simulink library "icc_lib_avg_path1_n1"  (R2018b)
settings: Solver=VariableStepAuto  StartTime=0.0  StopTime=10.0  RelTol=1e-3
undefined symbols (not defined in the file or in its folder): icc_lib_avg_path, path1
libraries: simulink x34, simulink_extras x8, $bdroot x2
(part 2 of 4)

== system icc_lib_avg_path1_n1/path_EGM1 ==
  mode1 : Inport
  mode2 : Inport  Port=2
  v1 : Inport  Port=3
  v2 : Inport  Port=4
  "xy1 " : Inport  Port=5
  xy2 : Inport  Port=6
  AND : Logic  IconShape=distinctive  AllPortsSameDT=off  OutDataTypeStr=boolean
  Data Type Conversion : DataTypeConversion  OutDataTypeStr=boolean
  Data Type Conversion1 : DataTypeConversion  OutDataTypeStr=boolean
  Delayed v1 : TransportDelay  DelayTime=0  BufferSize=200704
  Delayed v2 : TransportDelay  DelayTime=0  BufferSize=200704
  Demux : Demux  Outputs=2
  Demux1 : Demux  Outputs=2
  Logical Operator1 : Logic  Operator=OR  AllPortsSameDT=off  OutDataTypeStr=boolean
  Logical Operator2 : Logic  Operator=OR  AllPortsSameDT=off  OutDataTypeStr=boolean
  Mux : Mux  Inputs=6
  Path : Stateflow chart  TreatAsAtomicUnit=on
  Relay switch1 : MultiPortSwitch  DataPortOrder=Zero-based contiguous  Inputs=2  zeroidx=on
  Relay switch2 : MultiPortSwitch  DataPortOrder=Zero-based contiguous  Inputs=2  zeroidx=on
  S-R Flip-Flop : simulink_extras/Flip Flops/S-R Flip-Flop  initial_condition=0
  S-R Flip-Flop1 : simulink_extras/Flip Flops/S-R Flip-Flop  initial_condition=0
  Terminator : Terminator
  Terminator1 : Terminator
  Transport Delay1 : TransportDelay  DelayTime=0.1
  Transport Delay2 : TransportDelay  DelayTime=0.1
  cell1 resting : simulink/Logic and Bit Operations/Compare To Constant  relop===  const=0  OutDataTypeStr=boolean
  cell1FinishR : simulink/Logic and Bit Operations/Compare To Constant  relop=>=  const=1  OutDataTypeStr=boolean
  cell2 resting : simulink/Logic and Bit Operations/Compare To Constant  relop===  const=0  OutDataTypeStr=boolean
  cell2FinishR : simulink/Logic and Bit Operations/Compare To Constant  relop=>=  const=1  OutDataTypeStr=boolean
  cell2FinishR1 : simulink/Logic and Bit Operations/Compare To Constant  relop=~=  const=0  OutDataTypeStr=boolean
  cell2FinishR2 : simulink/Logic and Bit Operations/Compare To Constant  relop=~=  const=4  OutDataTypeStr=boolean
  zero : Constant  Value=-67.6
  zero1 : Constant  Value=-67.6
  relay_1 : Outport
  relay_2 : Outport  Port=2
  egm : Outport  Port=3
  wires:
  Data Type Conversion1/1 -> S-R Flip-Flop1/1
  Data Type Conversion/1 -> S-R Flip-Flop/1
  mode1/1 -> cell1FinishR/1, Transport Delay1/1, Path/1(mode1)
  Transport Delay2/1 -> Path/4(mdelay2), cell2 resting/1
  cell1FinishR/1 -> Logical Operator2/1
  Logical Operator2/1 -> S-R Flip-Flop1/2
  cell2 resting/1 -> Logical Operator2/2
  cell1 resting/1 -> Logical Operator1/2
  AND/1 -> Logical Operator1/1
  Logical Operator1/1 -> S-R Flip-Flop/2
  Relay switch2/1 -> relay_2/1
  S-R Flip-Flop1/2 -> Terminator1/1
  v1/1 -> Delayed v1/1
  Path/1(relay1) -> Data Type Conversion/1
  Delayed v1/1 -> Relay switch1/3
  S-R Flip-Flop1/1 -> Relay switch2/1
  Path/2(relay2) -> Data Type Conversion1/1
  v2/1 -> Delayed v2/1
  zero1/1 -> Relay switch2/2
  zero/1 -> Relay switch1/2
  S-R Flip-Flop/2 -> Terminator/1
  S-R Flip-Flop/1 -> Relay switch1/1
  Relay switch1/1 -> relay_1/1
  Delayed v2/1 -> Relay switch2/3
  mode2/1 -> cell2FinishR2/1, cell2FinishR1/1, Path/3(mode2), Transport Delay2/1
  Transport Delay1/1 -> Path/2(mdelay1), cell1 resting/1
  cell2FinishR1/1 -> AND/2
  cell2FinishR2/1 -> AND/1
  "xy1 "/1 -> Demux/1
  Demux/1 -> [x1]
  Demux/2 -> [y1]
  Mux/1 -> egm/1
  Path/3(t1) -> [t1]
  Path/4(t2) -> [t2]
  [t1] -> Mux/1
  [t2] -> Mux/2
  [x1] -> Mux/3
  [y1] -> Mux/4
  xy2/1 -> Demux1/1
  Demux1/1 -> [x2]
  Demux1/2 -> [y2]
  [y2] -> Mux/6
  [x2] -> Mux/5

== system icc_lib_avg_path1_n1/ICC /ODE ==
  q : Inport
  vreset : Inport  Port=2
  d0 : Inport  Port=3
  d1 : Inport  Port=4
  d2 : Inport  Port=5
  d3 : Inport  Port=6
  reset : Inport  Port=7
  IC : InitialCondition  Value=0
  Memory1 : Memory
  Multiport Switch1 : MultiPortSwitch  DataPortOrder=Zero-based contiguous  Inputs=6  zeroidx=on
  Switch Case : SwitchCase  CaseConditions={0,1,2,3,4,5}  ShowDefaultCase=off
  q0 : Subsystem  TreatAsAtomicUnit=on
  q1 : Subsystem  TreatAsAtomicUnit=on
  q2 : Subsystem  TreatAsAtomicUnit=on
  q3 : Subsystem  TreatAsAtomicUnit=on
  vt_0 : Outport
  wires:
  Multiport Switch1/1 -> Memory1/1
  IC/1 -> [vreset]
  vreset/1 -> IC/1
  reset/1 -> [reset]
  q/1 -> [q]
  q1/1(v) -> [pulse1]
  [q] -> Multiport Switch1/1
  [q] -> Switch Case/1
  [q1] -> q1/Action
  [reset] -> q1/1(reset)
  q2/1(v) -> [v2]
  d2/1 -> q2/3(d)
  [q2] -> q2/Action
  [vreset] -> q2/2(vreset)
  q3/1(v) -> [v3]
  d3/1 -> q3/3(d)
  [reset] -> q3/1(reset)
  [vreset] -> q3/2(vreset)
  q0/1(pulse) -> [v0]
  d0/1 -> q0/3(d)
  [reset] -> q0/1(reset)
  [vreset] -> q0/2(vreset)
  [q3] -> q3/Action
  [q0] -> q0/Action
  Memory1/1 -> vt_0/1
  [v0] -> Multiport Switch1/2
  [pulse1] -> Multiport Switch1/3
  [v2] -> Multiport Switch1/4
  [v3] -> Multiport Switch1/5
  [reset] -> q2/1(reset)
  [vreset] -> q1/2(vreset)
  d1/1 -> q1/3(d)
  Switch Case/1 -> [q0]
  Switch Case/2 -> [q1]
  Switch Case/3 -> [q2]
  Switch Case/4 -> [q3]

== system icc_lib_avg_path1_n1/ICC-multi/ODE ==
  q : Inport
  vreset : Inport  Port=2
  d0 : Inport  Port=3
  d1 : Inport  Port=4
  d2 : Inport  Port=5
  d3 : Inport  Port=6
  reset : Inport  Port=7
  IC : InitialCondition  Value=0
  Memory1 : Memory
  Multiport Switch1 : MultiPortSwitch  DataPortOrder=Zero-based contiguous  Inputs=6  zeroidx=on
  Switch Case : SwitchCase  CaseConditions={0,1,2,3,4,5}  ShowDefaultCase=off
  q0 : Subsystem  TreatAsAtomicUnit=on
  q1 : Subsystem  TreatAsAtomicUnit=on
  q2 : Subsystem  TreatAsAtomicUnit=on
  q3 : Subsystem  TreatAsAtomicUnit=on
  vt_0 : Outport
  wires:
  Switch Case/4 -> [q3]
  Switch Case/3 -> [q2]
  Switch Case/2 -> [q1]
  Switch Case/1 -> [q0]
  d1/1 -> q1/3(d)
  [vreset] -> q1/2(vreset)
  [reset] -> q2/1(reset)
  [v3] -> Multiport Switch1/5
  [v2] -> Multiport Switch1/4
  [pulse1] -> Multiport Switch1/3
  [v0] -> Multiport Switch1/2
  Memory1/1 -> vt_0/1
  [q0] -> q0/Action
  [q3] -> q3/Action
  [vreset] -> q0/2(vreset)
  [reset] -> q0/1(reset)
  d0/1 -> q0/3(d)
  q0/1(pulse) -> [v0]
  [vreset] -> q3/2(vreset)
  [reset] -> q3/1(reset)
  d3/1 -> q3/3(d)
  q3/1(v) -> [v3]
  [vreset] -> q2/2(vreset)
  [q2] -> q2/Action
  d2/1 -> q2/3(d)
  q2/1(v) -> [v2]
  [reset] -> q1/1(reset)
  [q1] -> q1/Action
  [q] -> Switch Case/1
  [q] -> Multiport Switch1/1
  q1/1(v) -> [pulse1]
  q/1 -> [q]
  reset/1 -> [reset]
  vreset/1 -> IC/1
  IC/1 -> [vreset]
  Multiport Switch1/1 -> Memory1/1

== system icc_lib_avg_path1_n1/ICC1/ODE ==
  q : Inport
  vreset : Inport  Port=2
  d0 : Inport  Port=3
  d1 : Inport  Port=4
  d2 : Inport  Port=5
  d3 : Inport  Port=6
  reset : Inport  Port=7
  IC : InitialCondition  Value=0
  Memory1 : Memory
  Multiport Switch1 : MultiPortSwitch  DataPortOrder=Zero-based contiguous  Inputs=6  zeroidx=on
  Switch Case : SwitchCase  CaseConditions={0,1,2,3,4,5}  ShowDefaultCase=off
  q0 : Subsystem  TreatAsAtomicUnit=on
  q1 : Subsystem  TreatAsAtomicUnit=on
  q2 : Subsystem  TreatAsAtomicUnit=on
  q3 : Subsystem  TreatAsAtomicUnit=on
  vt_0 : Outport
  wires:
  Switch Case/4 -> [q3]
  Switch Case/3 -> [q2]
  Switch Case/2 -> [q1]
  Switch Case/1 -> [q0]
  d1/1 -> q1/3(d)
  [vreset] -> q1/2(vreset)
  [reset] -> q2/1(reset)
  [v3] -> Multiport Switch1/5
  [v2] -> Multiport Switch1/4
  [pulse1] -> Multiport Switch1/3
  [v0] -> Multiport Switch1/2
  Memory1/1 -> vt_0/1
  [q0] -> q0/Action
  [q3] -> q3/Action
  [vreset] -> q0/2(vreset)
  [reset] -> q0/1(reset)
  d0/1 -> q0/3(d)
  q0/1(pulse) -> [v0]
  [vreset] -> q3/2(vreset)
  [reset] -> q3/1(reset)
  d3/1 -> q3/3(d)
  q3/1(v) -> [v3]
  [vreset] -> q2/2(vreset)
  [q2] -> q2/Action
  d2/1 -> q2/3(d)
  q2/1(v) -> [v2]
  [reset] -> q1/1(reset)
  [q1] -> q1/Action
  [q] -> Switch Case/1
  [q] -> Multiport Switch1/1
  q1/1(v) -> [pulse1]
  q/1 -> [q]
  reset/1 -> [reset]
  vreset/1 -> IC/1
  IC/1 -> [vreset]
  Multiport Switch1/1 -> Memory1/1

== system icc_lib_avg_path1_n1/ICC1_egm/ODE ==
  q : Inport
  vreset : Inport  Port=2
  d0 : Inport  Port=3
  d1 : Inport  Port=4
  d2 : Inport  Port=5
  d3 : Inport  Port=6
  reset : Inport  Port=7
  IC : InitialCondition  Value=0
  Memory1 : Memory
  Multiport Switch1 : MultiPortSwitch  DataPortOrder=Zero-based contiguous  Inputs=6  zeroidx=on
  Switch Case : SwitchCase  CaseConditions={0,1,2,3,4,5}  ShowDefaultCase=off
  q0 : Subsystem  TreatAsAtomicUnit=on
  q1 : Subsystem  TreatAsAtomicUnit=on
  q2 : Subsystem  TreatAsAtomicUnit=on
  q3 : Subsystem  TreatAsAtomicUnit=on
  vt_0 : Outport
  wires:
  Switch Case/4 -> [q3]
  Switch Case/3 -> [q2]
  Switch Case/2 -> [q1]
  Switch Case/1 -> [q0]
  d1/1 -> q1/3(d)
  [vreset] -> q1/2(vreset)
  [reset] -> q2/1(reset)
  [v3] -> Multiport Switch1/5
  [v2] -> Multiport Switch1/4
  [pulse1] -> Multiport Switch1/3
  [v0] -> Multiport Switch1/2
  Memory1/1 -> vt_0/1
  [q0] -> q0/Action
  [q3] -> q3/Action
  [vreset] -> q0/2(vreset)
  [reset] -> q0/1(reset)
  d0/1 -> q0/3(d)
  q0/1(pulse) -> [v0]
  [vreset] -> q3/2(vreset)
  [reset] -> q3/1(reset)
  d3/1 -> q3/3(d)
  q3/1(v) -> [v3]
  [vreset] -> q2/2(vreset)
  [q2] -> q2/Action
  d2/1 -> q2/3(d)
  q2/1(v) -> [v2]
  [reset] -> q1/1(reset)
  [q1] -> q1/Action
  [q] -> Switch Case/1
  [q] -> Multiport Switch1/1
  q1/1(v) -> [pulse1]
  q/1 -> [q]
  reset/1 -> [reset]
  vreset/1 -> IC/1
  IC/1 -> [vreset]
  Multiport Switch1/1 -> Memory1/1

== system icc_lib_avg_path1_n1/ICC1_egm_b/ODE ==
  q : Inport
  vreset : Inport  Port=2
  d0 : Inport  Port=3
  d1 : Inport  Port=4
  d2 : Inport  Port=5
  d3 : Inport  Port=6
  reset : Inport  Port=7
  IC : InitialCondition  Value=0
  Memory1 : Memory
  Multiport Switch1 : MultiPortSwitch  DataPortOrder=Zero-based contiguous  Inputs=6  zeroidx=on
  Switch Case : SwitchCase  CaseConditions={0,1,2,3,4,5}  ShowDefaultCase=off
  q0 : Subsystem  TreatAsAtomicUnit=on
  q1 : Subsystem  TreatAsAtomicUnit=on
  q2 : Subsystem  TreatAsAtomicUnit=on
  q3 : Subsystem  TreatAsAtomicUnit=on
  vt_0 : Outport
  wires:
  Switch Case/4 -> [q3]
  Switch Case/3 -> [q2]
  Switch Case/2 -> [q1]
  Switch Case/1 -> [q0]
  d1/1 -> q1/3(d)
  [vreset] -> q1/2(vreset)
  [reset] -> q2/1(reset)
  [v3] -> Multiport Switch1/5
  [v2] -> Multiport Switch1/4
  [pulse1] -> Multiport Switch1/3
  [v0] -> Multiport Switch1/2
  Memory1/1 -> vt_0/1
  [q0] -> q0/Action
  [q3] -> q3/Action
  [vreset] -> q0/2(vreset)
  [reset] -> q0/1(reset)
  d0/1 -> q0/3(d)
  q0/1(pulse) -> [v0]
  [vreset] -> q3/2(vreset)
  [reset] -> q3/1(reset)
  d3/1 -> q3/3(d)
  q3/1(v) -> [v3]
  [vreset] -> q2/2(vreset)
  [q2] -> q2/Action
  d2/1 -> q2/3(d)
  q2/1(v) -> [v2]
  [reset] -> q1/1(reset)
  [q1] -> q1/Action
  [q] -> Switch Case/1
  [q] -> Multiport Switch1/1
  q1/1(v) -> [pulse1]
  q/1 -> [q]
  reset/1 -> [reset]
  vreset/1 -> IC/1
  IC/1 -> [vreset]
  Multiport Switch1/1 -> Memory1/1

== system icc_lib_avg_path1_n1/ICC4/ODE ==
  q : Inport
  vreset : Inport  Port=2
  d0 : Inport  Port=3
  d1 : Inport  Port=4
  d2 : Inport  Port=5
  d3 : Inport  Port=6
  reset : Inport  Port=7
  IC : InitialCondition  Value=0
  Memory1 : Memory
  Multiport Switch1 : MultiPortSwitch  DataPortOrder=Zero-based contiguous  Inputs=6  zeroidx=on
  Switch Case : SwitchCase  CaseConditions={0,1,2,3,4,5}  ShowDefaultCase=off
  q0 : Subsystem  TreatAsAtomicUnit=on
  q1 : Subsystem  TreatAsAtomicUnit=on
  q2 : Subsystem  TreatAsAtomicUnit=on
  q3 : Subsystem  TreatAsAtomicUnit=on
  vt_0 : Outport
  wires:
  Switch Case/4 -> [q3]
  Switch Case/3 -> [q2]
  Switch Case/2 -> [q1]
  Switch Case/1 -> [q0]
  d1/1 -> q1/3(d)
  [vreset] -> q1/2(vreset)
  [reset] -> q2/1(reset)
  [v3] -> Multiport Switch1/5
  [v2] -> Multiport Switch1/4
  [pulse1] -> Multiport Switch1/3
  [v0] -> Multiport Switch1/2
  Memory1/1 -> vt_0/1
  [q0] -> q0/Action
  [q3] -> q3/Action
  [vreset] -> q0/2(vreset)
  [reset] -> q0/1(reset)
  d0/1 -> q0/3(d)
  q0/1(pulse) -> [v0]
  [vreset] -> q3/2(vreset)
  [reset] -> q3/1(reset)
  d3/1 -> q3/3(d)
  q3/1(v) -> [v3]
  [vreset] -> q2/2(vreset)
  [q2] -> q2/Action
  d2/1 -> q2/3(d)
  q2/1(v) -> [v2]
  [reset] -> q1/1(reset)
  [q1] -> q1/Action
  [q] -> Switch Case/1
  [q] -> Multiport Switch1/1
  q1/1(v) -> [pulse1]
  q/1 -> [q]
  reset/1 -> [reset]
  vreset/1 -> IC/1
  IC/1 -> [vreset]
  Multiport Switch1/1 -> Memory1/1

== system icc_lib_avg_path1_n1/ICC4_egm/ODE ==
  q : Inport
  vreset : Inport  Port=2
  d0 : Inport  Port=3
  d1 : Inport  Port=4
  d2 : Inport  Port=5
  d3 : Inport  Port=6
  reset : Inport  Port=7
  IC : InitialCondition  Value=0
  Memory1 : Memory
  Multiport Switch1 : MultiPortSwitch  DataPortOrder=Zero-based contiguous  Inputs=6  zeroidx=on
  Switch Case : SwitchCase  CaseConditions={0,1,2,3,4,5}  ShowDefaultCase=off
  q0 : Subsystem  TreatAsAtomicUnit=on
  q1 : Subsystem  TreatAsAtomicUnit=on
  q2 : Subsystem  TreatAsAtomicUnit=on
  q3 : Subsystem  TreatAsAtomicUnit=on
  vt_0 : Outport
  wires:
  Switch Case/4 -> [q3]
  Switch Case/3 -> [q2]
  Switch Case/2 -> [q1]
  Switch Case/1 -> [q0]
  d1/1 -> q1/3(d)
  [vreset] -> q1/2(vreset)
  [reset] -> q2/1(reset)
  [v3] -> Multiport Switch1/5
  [v2] -> Multiport Switch1/4
  [pulse1] -> Multiport Switch1/3
  [v0] -> Multiport Switch1/2
  Memory1/1 -> vt_0/1
  [q0] -> q0/Action
  [q3] -> q3/Action
  [vreset] -> q0/2(vreset)
  [reset] -> q0/1(reset)
  d0/1 -> q0/3(d)
  q0/1(pulse) -> [v0]
  [vreset] -> q3/2(vreset)
  [reset] -> q3/1(reset)
  d3/1 -> q3/3(d)
  q3/1(v) -> [v3]
  [vreset] -> q2/2(vreset)
  [q2] -> q2/Action
  d2/1 -> q2/3(d)
  q2/1(v) -> [v2]
  [reset] -> q1/1(reset)
  [q1] -> q1/Action
  [q] -> Switch Case/1
  [q] -> Multiport Switch1/1
  q1/1(v) -> [pulse1]
  q/1 -> [q]
  reset/1 -> [reset]
  vreset/1 -> IC/1
  IC/1 -> [vreset]
  Multiport Switch1/1 -> Memory1/1

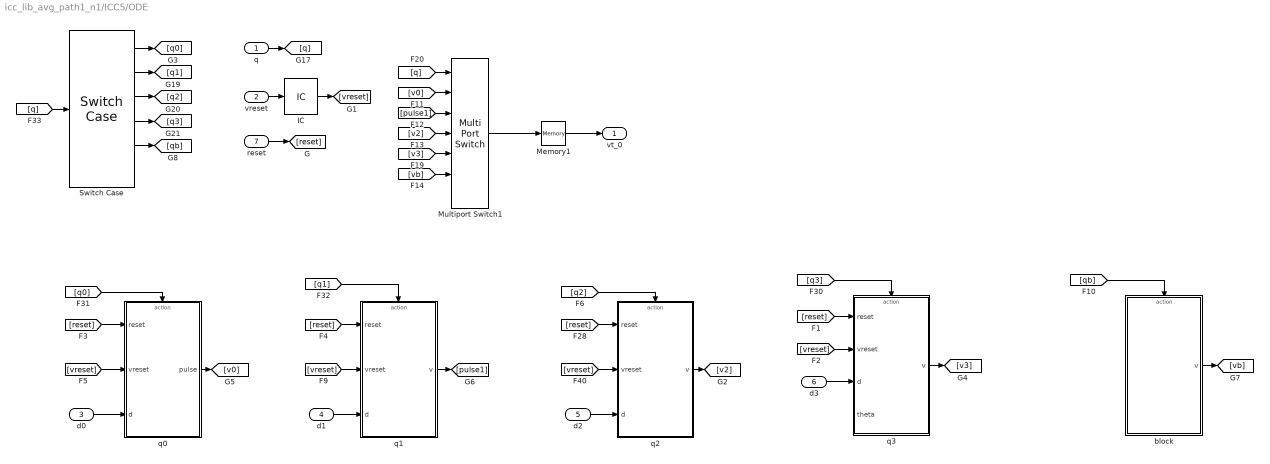
== system icc_lib_avg_path1_n1/ICC5/ODE ==
  q : Inport
  vreset : Inport  Port=2
  d0 : Inport  Port=3
  d1 : Inport  Port=4
  d2 : Inport  Port=5
  d3 : Inport  Port=6
  reset : Inport  Port=7
  IC : InitialCondition  Value=0
  Memory1 : Memory
  Multiport Switch1 : MultiPortSwitch  DataPortOrder=Zero-based contiguous  Inputs=6  zeroidx=on
  Switch Case : SwitchCase  CaseConditions={0,1,2,3,4,5}  ShowDefaultCase=off
  block : Subsystem  TreatAsAtomicUnit=on
  q0 : Subsystem  TreatAsAtomicUnit=on
  q1 : Subsystem  TreatAsAtomicUnit=on
  q2 : Subsystem  TreatAsAtomicUnit=on
  q3 : Subsystem  TreatAsAtomicUnit=on
  vt_0 : Outport
  wires:
  Switch Case/4 -> [q3]
  Switch Case/3 -> [q2]
  Switch Case/2 -> [q1]
  Switch Case/1 -> [q0]
  d1/1 -> q1/3(d)
  [vreset] -> q1/2(vreset)
  [reset] -> q2/1(reset)
  [v3] -> Multiport Switch1/5
  [v2] -> Multiport Switch1/4
  [pulse1] -> Multiport Switch1/3
  [v0] -> Multiport Switch1/2
  Memory1/1 -> vt_0/1
  [q0] -> q0/Action
  [q3] -> q3/Action
  [vreset] -> q0/2(vreset)
  [reset] -> q0/1(reset)
  d0/1 -> q0/3(d)
  q0/1(pulse) -> [v0]
  [vreset] -> q3/2(vreset)
  [reset] -> q3/1(reset)
  d3/1 -> q3/3(d)
  q3/1(v) -> [v3]
  [vreset] -> q2/2(vreset)
  [q2] -> q2/Action
  d2/1 -> q2/3(d)
  q2/1(v) -> [v2]
  [reset] -> q1/1(reset)
  [q1] -> q1/Action
  [q] -> Switch Case/1
  [q] -> Multiport Switch1/1
  q1/1(v) -> [pulse1]
  q/1 -> [q]
  reset/1 -> [reset]
  vreset/1 -> IC/1
  IC/1 -> [vreset]
  Multiport Switch1/1 -> Memory1/1
  [qb] -> block/Action
  block/1(v) -> [vb]
  Switch Case/5 -> [qb]
  [vb] -> Multiport Switch1/6

== system icc_lib_avg_path1_n1/ICC5_egm/ODE ==
  q : Inport
  vreset : Inport  Port=2
  d0 : Inport  Port=3
  d1 : Inport  Port=4
  d2 : Inport  Port=5
  d3 : Inport  Port=6
  reset : Inport  Port=7
  IC : InitialCondition  Value=0
  Memory1 : Memory
  Multiport Switch1 : MultiPortSwitch  DataPortOrder=Zero-based contiguous  Inputs=6  zeroidx=on
  Switch Case : SwitchCase  CaseConditions={0,1,2,3,4,5}  ShowDefaultCase=off
  block : Subsystem  TreatAsAtomicUnit=on
  q0 : Subsystem  TreatAsAtomicUnit=on
  q1 : Subsystem  TreatAsAtomicUnit=on
  q2 : Subsystem  TreatAsAtomicUnit=on
  q3 : Subsystem  TreatAsAtomicUnit=on
  vt_0 : Outport
  wires:
  Switch Case/4 -> [q3]
  Switch Case/3 -> [q2]
  Switch Case/2 -> [q1]
  Switch Case/1 -> [q0]
  d1/1 -> q1/3(d)
  [vreset] -> q1/2(vreset)
  [reset] -> q2/1(reset)
  [v3] -> Multiport Switch1/5
  [v2] -> Multiport Switch1/4
  [pulse1] -> Multiport Switch1/3
  [v0] -> Multiport Switch1/2
  Memory1/1 -> vt_0/1
  [q0] -> q0/Action
  [q3] -> q3/Action
  [vreset] -> q0/2(vreset)
  [reset] -> q0/1(reset)
  d0/1 -> q0/3(d)
  q0/1(pulse) -> [v0]
  [vreset] -> q3/2(vreset)
  [reset] -> q3/1(reset)
  d3/1 -> q3/3(d)
  q3/1(v) -> [v3]
  [vreset] -> q2/2(vreset)
  [q2] -> q2/Action
  d2/1 -> q2/3(d)
  q2/1(v) -> [v2]
  [reset] -> q1/1(reset)
  [q1] -> q1/Action
  [q] -> Switch Case/1
  [q] -> Multiport Switch1/1
  q1/1(v) -> [pulse1]
  q/1 -> [q]
  reset/1 -> [reset]
  vreset/1 -> IC/1
  IC/1 -> [vreset]
  Multiport Switch1/1 -> Memory1/1
  [qb] -> block/Action
  block/1(v) -> [vb]
  Switch Case/5 -> [qb]
  [vb] -> Multiport Switch1/6

== system icc_lib_avg_path1_n1/ICC6/ODE ==
  q : Inport
  vreset : Inport  Port=2
  d0 : Inport  Port=3
  d1 : Inport  Port=4
  d2 : Inport  Port=5
  d3 : Inport  Port=6
  reset : Inport  Port=7
  IC : InitialCondition  Value=0
  Memory1 : Memory
  Multiport Switch1 : MultiPortSwitch  DataPortOrder=Zero-based contiguous  Inputs=6  zeroidx=on
  Switch Case : SwitchCase  CaseConditions={0,1,2,3,4,5}  ShowDefaultCase=off
  block : Subsystem  TreatAsAtomicUnit=on
  q0 : Subsystem  TreatAsAtomicUnit=on
  q1 : Subsystem  TreatAsAtomicUnit=on
  q2 : Subsystem  TreatAsAtomicUnit=on
  q3 : Subsystem  TreatAsAtomicUnit=on
  vt_0 : Outport
  wires:
  Switch Case/4 -> [q3]
  Switch Case/3 -> [q2]
  Switch Case/2 -> [q1]
  Switch Case/1 -> [q0]
  d1/1 -> q1/3(d)
  [vreset] -> q1/2(vreset)
  [reset] -> q2/1(reset)
  [v3] -> Multiport Switch1/5
  [v2] -> Multiport Switch1/4
  [pulse1] -> Multiport Switch1/3
  [v0] -> Multiport Switch1/2
  Memory1/1 -> vt_0/1
  [q0] -> q0/Action
  [q3] -> q3/Action
  [vreset] -> q0/2(vreset)
  [reset] -> q0/1(reset)
  d0/1 -> q0/3(d)
  q0/1(pulse) -> [v0]
  [vreset] -> q3/2(vreset)
  [reset] -> q3/1(reset)
  d3/1 -> q3/3(d)
  q3/1(v) -> [v3]
  [vreset] -> q2/2(vreset)
  [q2] -> q2/Action
  d2/1 -> q2/3(d)
  q2/1(v) -> [v2]
  [reset] -> q1/1(reset)
  [q1] -> q1/Action
  [q] -> Switch Case/1
  [q] -> Multiport Switch1/1
  q1/1(v) -> [pulse1]
  q/1 -> [q]
  reset/1 -> [reset]
  vreset/1 -> IC/1
  IC/1 -> [vreset]
  Multiport Switch1/1 -> Memory1/1
  [qb] -> block/Action
  block/1(v) -> [vb]
  Switch Case/5 -> [qb]
  [vb] -> Multiport Switch1/6

== system icc_lib_avg_path1_n1/ICC6_egm/ODE ==
  q : Inport
  vreset : Inport  Port=2
  d0 : Inport  Port=3
  d1 : Inport  Port=4
  d2 : Inport  Port=5
  d3 : Inport  Port=6
  reset : Inport  Port=7
  IC : InitialCondition  Value=0
  Memory1 : Memory
  Multiport Switch1 : MultiPortSwitch  DataPortOrder=Zero-based contiguous  Inputs=6  zeroidx=on
  Switch Case : SwitchCase  CaseConditions={0,1,2,3,4,5}  ShowDefaultCase=off
  block : Subsystem  TreatAsAtomicUnit=on
  q0 : Subsystem  TreatAsAtomicUnit=on
  q1 : Subsystem  TreatAsAtomicUnit=on
  q2 : Subsystem  TreatAsAtomicUnit=on
  q3 : Subsystem  TreatAsAtomicUnit=on
  vt_0 : Outport
  wires:
  [vb] -> Multiport Switch1/6
  Switch Case/5 -> [qb]
  block/1(v) -> [vb]
  [qb] -> block/Action
  Multiport Switch1/1 -> Memory1/1
  IC/1 -> [vreset]
  vreset/1 -> IC/1
  reset/1 -> [reset]
  q/1 -> [q]
  q1/1(v) -> [pulse1]
  [q] -> Multiport Switch1/1
  [q] -> Switch Case/1
  [q1] -> q1/Action
  [reset] -> q1/1(reset)
  q2/1(v) -> [v2]
  d2/1 -> q2/3(d)
  [q2] -> q2/Action
  [vreset] -> q2/2(vreset)
  q3/1(v) -> [v3]
  d3/1 -> q3/3(d)
  [reset] -> q3/1(reset)
  [vreset] -> q3/2(vreset)
  q0/1(pulse) -> [v0]
  d0/1 -> q0/3(d)
  [reset] -> q0/1(reset)
  [vreset] -> q0/2(vreset)
  [q3] -> q3/Action
  [q0] -> q0/Action
  Memory1/1 -> vt_0/1
  [v0] -> Multiport Switch1/2
  [pulse1] -> Multiport Switch1/3
  [v2] -> Multiport Switch1/4
  [v3] -> Multiport Switch1/5
  [reset] -> q2/1(reset)
  [vreset] -> q1/2(vreset)
  d1/1 -> q1/3(d)
  Switch Case/1 -> [q0]
  Switch Case/2 -> [q1]
  Switch Case/3 -> [q2]
  Switch Case/4 -> [q3]

== system icc_lib_avg_path1_n1/ICC /ODE/q0 ==
  reset : Inport
  vreset : Inport  Port=2
  d : Inport  Port=3
  Action Port : ActionPort  InitializeStates=reset
  Integrator1 : Integrator  ExternalReset=either  InitialConditionSource=external  InitialCondition=20
  pulse : Outport
  wires:
  vreset/1 -> Integrator1/3
  reset/1 -> Integrator1/2
  d/1 -> Integrator1/1
  Integrator1/1 -> pulse/1

== system icc_lib_avg_path1_n1/ICC /ODE/q1 ==
  reset : Inport
  vreset : Inport  Port=2
  d : Inport  Port=3
  Action Port : ActionPort  InitializeStates=reset
  Integrator1 : Integrator  ExternalReset=either  InitialConditionSource=external  InitialCondition=20
  v : Outport
  wires:
  vreset/1 -> Integrator1/3
  reset/1 -> Integrator1/2
  Integrator1/1 -> v/1
  d/1 -> Integrator1/1

== system icc_lib_avg_path1_n1/ICC /ODE/q2 ==
  reset : Inport
  vreset : Inport  Port=2
  d : Inport  Port=3
  Action Port : ActionPort  InitializeStates=reset
  Integrator1 : Integrator  ExternalReset=either  InitialConditionSource=external  InitialCondition=20
  v : Outport
  wires:
  Integrator1/1 -> v/1
  reset/1 -> Integrator1/2
  vreset/1 -> Integrator1/3
  d/1 -> Integrator1/1

== system icc_lib_avg_path1_n1/ICC /ODE/q3 ==
  reset : Inport
  vreset : Inport  Port=2
  d : Inport  Port=3
  theta : Inport  Port=4
  Action Port : ActionPort  InitializeStates=reset
  C : Constant  Value=-1
  Integrator1 : Integrator  ExternalReset=either  InitialConditionSource=external  InitialCondition=20
  Math Function : Math  SaturateOnIntegerOverflow=on
  Product1 : Product
  Product2 : Product
  v : Outport
  wires:
  vreset/1 -> Integrator1/3
  reset/1 -> Integrator1/2
  Integrator1/1 -> v/1
  Math Function/1 -> Product1/2
  theta/1 -> Product2/1
  Product1/1 -> ?
  C/1 -> Product2/2
  Product2/1 -> Math Function/1
  d/1 -> Integrator1/1

== system icc_lib_avg_path1_n1/ICC-multi/ODE/q0 ==
  reset : Inport
  vreset : Inport  Port=2
  d : Inport  Port=3
  Action Port : ActionPort  InitializeStates=reset
  Integrator1 : Integrator  ExternalReset=either  InitialConditionSource=external  InitialCondition=20
  pulse : Outport
  wires:
  Integrator1/1 -> pulse/1
  d/1 -> Integrator1/1
  reset/1 -> Integrator1/2
  vreset/1 -> Integrator1/3

== system icc_lib_avg_path1_n1/ICC-multi/ODE/q1 ==
  reset : Inport
  vreset : Inport  Port=2
  d : Inport  Port=3
  Action Port : ActionPort  InitializeStates=reset
  Integrator1 : Integrator  ExternalReset=either  InitialConditionSource=external  InitialCondition=20
  v : Outport
  wires:
  d/1 -> Integrator1/1
  Integrator1/1 -> v/1
  reset/1 -> Integrator1/2
  vreset/1 -> Integrator1/3

== system icc_lib_avg_path1_n1/ICC-multi/ODE/q2 ==
  reset : Inport
  vreset : Inport  Port=2
  d : Inport  Port=3
  Action Port : ActionPort  InitializeStates=reset
  Integrator1 : Integrator  ExternalReset=either  InitialConditionSource=external  InitialCondition=20
  v : Outport
  wires:
  d/1 -> Integrator1/1
  vreset/1 -> Integrator1/3
  reset/1 -> Integrator1/2
  Integrator1/1 -> v/1

== system icc_lib_avg_path1_n1/ICC-multi/ODE/q3 ==
  reset : Inport
  vreset : Inport  Port=2
  d : Inport  Port=3
  theta : Inport  Port=4
  Action Port : ActionPort  InitializeStates=reset
  C : Constant  Value=-1
  Integrator1 : Integrator  ExternalReset=either  InitialConditionSource=external  InitialCondition=20
  Math Function : Math  SaturateOnIntegerOverflow=on
  Product1 : Product
  Product2 : Product
  v : Outport
  wires:
  d/1 -> Integrator1/1
  Product2/1 -> Math Function/1
  C/1 -> Product2/2
  Product1/1 -> ?
  theta/1 -> Product2/1
  Math Function/1 -> Product1/2
  Integrator1/1 -> v/1
  reset/1 -> Integrator1/2
  vreset/1 -> Integrator1/3

== system icc_lib_avg_path1_n1/ICC1/ODE/q0 ==
  reset : Inport
  vreset : Inport  Port=2
  d : Inport  Port=3
  Action Port : ActionPort  InitializeStates=reset
  Integrator1 : Integrator  ExternalReset=either  InitialConditionSource=external  InitialCondition=20
  pulse : Outport
  wires:
  Integrator1/1 -> pulse/1
  d/1 -> Integrator1/1
  reset/1 -> Integrator1/2
  vreset/1 -> Integrator1/3

== system icc_lib_avg_path1_n1/ICC1/ODE/q1 ==
  reset : Inport
  vreset : Inport  Port=2
  d : Inport  Port=3
  Action Port : ActionPort  InitializeStates=reset
  Display : Display
  Display1 : Display
  Integrator1 : Integrator  ExternalReset=either  InitialConditionSource=external  InitialCondition=20  LimitOutput=on  UpperSaturationLimit=-24.105
  Scope : Scope
  v : Outport
  wires:
  d/1 -> Integrator1/1
  Integrator1/1 -> Display/1, Scope/1, v/1
  reset/1 -> Integrator1/2
  vreset/1 -> Display1/1, Integrator1/3

== system icc_lib_avg_path1_n1/ICC1/ODE/q2 ==
  reset : Inport
  vreset : Inport  Port=2
  d : Inport  Port=3
  Action Port : ActionPort  InitializeStates=reset
  Integrator1 : Integrator  ExternalReset=either  InitialConditionSource=external  InitialCondition=20
  v : Outport
  wires:
  d/1 -> Integrator1/1
  vreset/1 -> Integrator1/3
  reset/1 -> Integrator1/2
  Integrator1/1 -> v/1

== system icc_lib_avg_path1_n1/ICC1/ODE/q3 ==
  reset : Inport
  vreset : Inport  Port=2
  d : Inport  Port=3
  theta : Inport  Port=4
  Action Port : ActionPort  InitializeStates=reset
  C : Constant  Value=-1
  Integrator1 : Integrator  ExternalReset=either  InitialConditionSource=external  InitialCondition=20  LimitOutput=on  LowerSaturationLimit=-67
  Math Function : Math  SaturateOnIntegerOverflow=on
  Product1 : Product
  Product2 : Product
  v : Outport
  wires:
  d/1 -> Integrator1/1
  Product2/1 -> Math Function/1
  C/1 -> Product2/2
  Product1/1 -> ?
  theta/1 -> Product2/1
  Math Function/1 -> Product1/2
  Integrator1/1 -> v/1
  reset/1 -> Integrator1/2
  vreset/1 -> Integrator1/3

== system icc_lib_avg_path1_n1/ICC1_egm/ODE/q0 ==
  reset : Inport
  vreset : Inport  Port=2
  d : Inport  Port=3
  Action Port : ActionPort  InitializeStates=reset
  Integrator1 : Integrator  ExternalReset=either  InitialConditionSource=external  InitialCondition=20
  pulse : Outport
  wires:
  Integrator1/1 -> pulse/1
  d/1 -> Integrator1/1
  reset/1 -> Integrator1/2
  vreset/1 -> Integrator1/3

== system icc_lib_avg_path1_n1/ICC1_egm/ODE/q1 ==
  reset : Inport
  vreset : Inport  Port=2
  d : Inport  Port=3
  Action Port : ActionPort  InitializeStates=reset
  Display : Display
  Display1 : Display
  Integrator1 : Integrator  ExternalReset=either  InitialConditionSource=external  InitialCondition=20  LimitOutput=on  UpperSaturationLimit=-24.105
  Scope : Scope
  v : Outport
  wires:
  d/1 -> Integrator1/1
  Integrator1/1 -> Display/1, Scope/1, v/1
  reset/1 -> Integrator1/2
  vreset/1 -> Display1/1, Integrator1/3

== system icc_lib_avg_path1_n1/ICC1_egm/ODE/q2 ==
  reset : Inport
  vreset : Inport  Port=2
  d : Inport  Port=3
  Action Port : ActionPort  InitializeStates=reset
  Integrator1 : Integrator  ExternalReset=either  InitialConditionSource=external  InitialCondition=20
  v : Outport
  wires:
  d/1 -> Integrator1/1
  vreset/1 -> Integrator1/3
  reset/1 -> Integrator1/2
  Integrator1/1 -> v/1

== system icc_lib_avg_path1_n1/ICC1_egm/ODE/q3 ==
  reset : Inport
  vreset : Inport  Port=2
  d : Inport  Port=3
  theta : Inport  Port=4
  Action Port : ActionPort  InitializeStates=reset
  C : Constant  Value=-1
  Integrator1 : Integrator  ExternalReset=either  InitialConditionSource=external  InitialCondition=20  LimitOutput=on  LowerSaturationLimit=-67
  Math Function : Math  SaturateOnIntegerOverflow=on
  Product1 : Product
  Product2 : Product
  v : Outport
  wires:
  d/1 -> Integrator1/1
  Product2/1 -> Math Function/1
  C/1 -> Product2/2
  Product1/1 -> ?
  theta/1 -> Product2/1
  Math Function/1 -> Product1/2
  Integrator1/1 -> v/1
  reset/1 -> Integrator1/2
  vreset/1 -> Integrator1/3

== system icc_lib_avg_path1_n1/ICC1_egm_b/ODE/q0 ==
  reset : Inport
  vreset : Inport  Port=2
  d : Inport  Port=3
  Action Port : ActionPort  InitializeStates=reset
  Integrator1 : Integrator  ExternalReset=either  InitialConditionSource=external  InitialCondition=20
  pulse : Outport
  wires:
  Integrator1/1 -> pulse/1
  d/1 -> Integrator1/1
  reset/1 -> Integrator1/2
  vreset/1 -> Integrator1/3

== system icc_lib_avg_path1_n1/ICC1_egm_b/ODE/q1 ==
  reset : Inport
  vreset : Inport  Port=2
  d : Inport  Port=3
  Action Port : ActionPort  InitializeStates=reset
  Display : Display
  Display1 : Display
  Integrator1 : Integrator  ExternalReset=either  InitialConditionSource=external  InitialCondition=20  LimitOutput=on  UpperSaturationLimit=-24.105
  Scope : Scope
  v : Outport
  wires:
  d/1 -> Integrator1/1
  Integrator1/1 -> Display/1, Scope/1, v/1
  reset/1 -> Integrator1/2
  vreset/1 -> Display1/1, Integrator1/3

== system icc_lib_avg_path1_n1/ICC1_egm_b/ODE/q2 ==
  reset : Inport
  vreset : Inport  Port=2
  d : Inport  Port=3
  Action Port : ActionPort  InitializeStates=reset
  Integrator1 : Integrator  ExternalReset=either  InitialConditionSource=external  InitialCondition=20
  v : Outport
  wires:
  d/1 -> Integrator1/1
  vreset/1 -> Integrator1/3
  reset/1 -> Integrator1/2
  Integrator1/1 -> v/1

== system icc_lib_avg_path1_n1/ICC1_egm_b/ODE/q3 ==
  reset : Inport
  vreset : Inport  Port=2
  d : Inport  Port=3
  theta : Inport  Port=4
  Action Port : ActionPort  InitializeStates=reset
  C : Constant  Value=-1
  Integrator1 : Integrator  ExternalReset=either  InitialConditionSource=external  InitialCondition=20  LimitOutput=on  LowerSaturationLimit=-67
  Math Function : Math  SaturateOnIntegerOverflow=on
  Product1 : Product
  Product2 : Product
  v : Outport
  wires:
  d/1 -> Integrator1/1
  Product2/1 -> Math Function/1
  C/1 -> Product2/2
  Product1/1 -> ?
  theta/1 -> Product2/1
  Math Function/1 -> Product1/2
  Integrator1/1 -> v/1
  reset/1 -> Integrator1/2
  vreset/1 -> Integrator1/3

== system icc_lib_avg_path1_n1/ICC4/ODE/q0 ==
  reset : Inport
  vreset : Inport  Port=2
  d : Inport  Port=3
  Action Port : ActionPort  InitializeStates=reset
  Integrator1 : Integrator  ExternalReset=either  InitialConditionSource=external  InitialCondition=20
  pulse : Outport
  wires:
  Integrator1/1 -> pulse/1
  d/1 -> Integrator1/1
  reset/1 -> Integrator1/2
  vreset/1 -> Integrator1/3

== system icc_lib_avg_path1_n1/ICC4/ODE/q1 ==
  reset : Inport
  vreset : Inport  Port=2
  d : Inport  Port=3
  Action Port : ActionPort  InitializeStates=reset
  Display : Display
  Display1 : Display
  Integrator1 : Integrator  ExternalReset=either  InitialConditionSource=external  InitialCondition=20  LimitOutput=on  UpperSaturationLimit=-24.105
  Scope : Scope
  v : Outport
  wires:
  d/1 -> Integrator1/1
  Integrator1/1 -> Display/1, Scope/1, v/1
  reset/1 -> Integrator1/2
  vreset/1 -> Display1/1, Integrator1/3

== system icc_lib_avg_path1_n1/ICC4/ODE/q2 ==
  reset : Inport
  vreset : Inport  Port=2
  d : Inport  Port=3
  Action Port : ActionPort  InitializeStates=reset
  Integrator1 : Integrator  ExternalReset=either  InitialConditionSource=external  InitialCondition=20
  v : Outport
  wires:
  d/1 -> Integrator1/1
  vreset/1 -> Integrator1/3
  reset/1 -> Integrator1/2
  Integrator1/1 -> v/1

== system icc_lib_avg_path1_n1/ICC4/ODE/q3 ==
  reset : Inport
  vreset : Inport  Port=2
  d : Inport  Port=3
  theta : Inport  Port=4
  Action Port : ActionPort  InitializeStates=reset
  C : Constant  Value=-1
  Integrator1 : Integrator  ExternalReset=either  InitialConditionSource=external  InitialCondition=20  LimitOutput=on  LowerSaturationLimit=-67
  Math Function : Math  SaturateOnIntegerOverflow=on
  Product1 : Product
  Product2 : Product
  v : Outport
  wires:
  d/1 -> Integrator1/1
  Product2/1 -> Math Function/1
  C/1 -> Product2/2
  Product1/1 -> ?
  theta/1 -> Product2/1
  Math Function/1 -> Product1/2
  Integrator1/1 -> v/1
  reset/1 -> Integrator1/2
  vreset/1 -> Integrator1/3

== system icc_lib_avg_path1_n1/ICC4_egm/ODE/q0 ==
  reset : Inport
  vreset : Inport  Port=2
  d : Inport  Port=3
  Action Port : ActionPort  InitializeStates=reset
  Integrator1 : Integrator  ExternalReset=either  InitialConditionSource=external  InitialCondition=20
  pulse : Outport
  wires:
  Integrator1/1 -> pulse/1
  d/1 -> Integrator1/1
  reset/1 -> Integrator1/2
  vreset/1 -> Integrator1/3

== system icc_lib_avg_path1_n1/ICC4_egm/ODE/q1 ==
  reset : Inport
  vreset : Inport  Port=2
  d : Inport  Port=3
  Action Port : ActionPort  InitializeStates=reset
  Display : Display
  Display1 : Display
  Integrator1 : Integrator  ExternalReset=either  InitialConditionSource=external  InitialCondition=20  LimitOutput=on  UpperSaturationLimit=-24.105
  Scope : Scope
  v : Outport
  wires:
  d/1 -> Integrator1/1
  Integrator1/1 -> Display/1, Scope/1, v/1
  reset/1 -> Integrator1/2
  vreset/1 -> Display1/1, Integrator1/3

== system icc_lib_avg_path1_n1/ICC4_egm/ODE/q2 ==
  reset : Inport
  vreset : Inport  Port=2
  d : Inport  Port=3
  Action Port : ActionPort  InitializeStates=reset
  Integrator1 : Integrator  ExternalReset=either  InitialConditionSource=external  InitialCondition=20
  v : Outport
  wires:
  d/1 -> Integrator1/1
  vreset/1 -> Integrator1/3
  reset/1 -> Integrator1/2
  Integrator1/1 -> v/1

== system icc_lib_avg_path1_n1/ICC4_egm/ODE/q3 ==
  reset : Inport
  vreset : Inport  Port=2
  d : Inport  Port=3
  theta : Inport  Port=4
  Action Port : ActionPort  InitializeStates=reset
  C : Constant  Value=-1
  Integrator1 : Integrator  ExternalReset=either  InitialConditionSource=external  InitialCondition=20  LimitOutput=on  LowerSaturationLimit=-67
  Math Function : Math  SaturateOnIntegerOverflow=on
  Product1 : Product
  Product2 : Product
  v : Outport
  wires:
  d/1 -> Integrator1/1
  Product2/1 -> Math Function/1
  C/1 -> Product2/2
  Product1/1 -> ?
  theta/1 -> Product2/1
  Math Function/1 -> Product1/2
  Integrator1/1 -> v/1
  reset/1 -> Integrator1/2
  vreset/1 -> Integrator1/3

== system icc_lib_avg_path1_n1/ICC5/ODE/block ==
  Action Port : ActionPort  InitializeStates=reset
  Constant : Constant  Value=-67.39
  v : Outport
  wires:
  Constant/1 -> v/1

== system icc_lib_avg_path1_n1/ICC5/ODE/q0 ==
  reset : Inport
  vreset : Inport  Port=2
  d : Inport  Port=3
  Action Port : ActionPort  InitializeStates=reset
  Integrator1 : Integrator  ExternalReset=either  InitialConditionSource=external  InitialCondition=20
  pulse : Outport
  wires:
  Integrator1/1 -> pulse/1
  d/1 -> Integrator1/1
  reset/1 -> Integrator1/2
  vreset/1 -> Integrator1/3

== system icc_lib_avg_path1_n1/ICC5/ODE/q1 ==
  reset : Inport
  vreset : Inport  Port=2
  d : Inport  Port=3
  Action Port : ActionPort  InitializeStates=reset
  Display : Display
  Display1 : Display
  Integrator1 : Integrator  ExternalReset=either  InitialConditionSource=external  InitialCondition=20  LimitOutput=on  UpperSaturationLimit=-24.105
  Scope : Scope
  v : Outport
  wires:
  d/1 -> Integrator1/1
  Integrator1/1 -> Display/1, Scope/1, v/1
  reset/1 -> Integrator1/2
  vreset/1 -> Display1/1, Integrator1/3

== system icc_lib_avg_path1_n1/ICC5/ODE/q2 ==
  reset : Inport
  vreset : Inport  Port=2
  d : Inport  Port=3
  Action Port : ActionPort  InitializeStates=reset
  Integrator1 : Integrator  ExternalReset=either  InitialConditionSource=external  InitialCondition=20
  v : Outport
  wires:
  d/1 -> Integrator1/1
  vreset/1 -> Integrator1/3
  reset/1 -> Integrator1/2
  Integrator1/1 -> v/1

== system icc_lib_avg_path1_n1/ICC5/ODE/q3 ==
  reset : Inport
  vreset : Inport  Port=2
  d : Inport  Port=3
  theta : Inport  Port=4
  Action Port : ActionPort  InitializeStates=reset
  C : Constant  Value=-1
  Integrator1 : Integrator  ExternalReset=either  InitialConditionSource=external  InitialCondition=20  LimitOutput=on  LowerSaturationLimit=-67
  Math Function : Math  SaturateOnIntegerOverflow=on
  Product1 : Product
  Product2 : Product
  v : Outport
  wires:
  d/1 -> Integrator1/1
  Product2/1 -> Math Function/1
  C/1 -> Product2/2
  Product1/1 -> ?
  theta/1 -> Product2/1
  Math Function/1 -> Product1/2
  Integrator1/1 -> v/1
  reset/1 -> Integrator1/2
  vreset/1 -> Integrator1/3

== system icc_lib_avg_path1_n1/ICC5_egm/ODE/block ==
  Action Port : ActionPort  InitializeStates=reset
  Constant : Constant  Value=-67.39
  v : Outport
  wires:
  Constant/1 -> v/1

== system icc_lib_avg_path1_n1/ICC5_egm/ODE/q0 ==
  reset : Inport
  vreset : Inport  Port=2
  d : Inport  Port=3
  Action Port : ActionPort  InitializeStates=reset
  Integrator1 : Integrator  ExternalReset=either  InitialConditionSource=external  InitialCondition=20
  pulse : Outport
  wires:
  Integrator1/1 -> pulse/1
  d/1 -> Integrator1/1
  reset/1 -> Integrator1/2
  vreset/1 -> Integrator1/3

== system icc_lib_avg_path1_n1/ICC5_egm/ODE/q1 ==
  reset : Inport
  vreset : Inport  Port=2
  d : Inport  Port=3
  Action Port : ActionPort  InitializeStates=reset
  Display : Display
  Display1 : Display
  Integrator1 : Integrator  ExternalReset=either  InitialConditionSource=external  InitialCondition=20  LimitOutput=on  UpperSaturationLimit=-24.105
  Scope : Scope
  v : Outport
  wires:
  d/1 -> Integrator1/1
  Integrator1/1 -> Display/1, Scope/1, v/1
  reset/1 -> Integrator1/2
  vreset/1 -> Display1/1, Integrator1/3

== system icc_lib_avg_path1_n1/ICC5_egm/ODE/q2 ==
  reset : Inport
  vreset : Inport  Port=2
  d : Inport  Port=3
  Action Port : ActionPort  InitializeStates=reset
  Integrator1 : Integrator  ExternalReset=either  InitialConditionSource=external  InitialCondition=20
  v : Outport
  wires:
  d/1 -> Integrator1/1
  vreset/1 -> Integrator1/3
  reset/1 -> Integrator1/2
  Integrator1/1 -> v/1

== system icc_lib_avg_path1_n1/ICC5_egm/ODE/q3 ==
  reset : Inport
  vreset : Inport  Port=2
  d : Inport  Port=3
  theta : Inport  Port=4
  Action Port : ActionPort  InitializeStates=reset
  C : Constant  Value=-1
  Integrator1 : Integrator  ExternalReset=either  InitialConditionSource=external  InitialCondition=20  LimitOutput=on  LowerSaturationLimit=-67
  Math Function : Math  SaturateOnIntegerOverflow=on
  Product1 : Product
  Product2 : Product
  v : Outport
  wires:
  d/1 -> Integrator1/1
  Product2/1 -> Math Function/1
  C/1 -> Product2/2
  Product1/1 -> ?
  theta/1 -> Product2/1
  Math Function/1 -> Product1/2
  Integrator1/1 -> v/1
  reset/1 -> Integrator1/2
  vreset/1 -> Integrator1/3

== system icc_lib_avg_path1_n1/ICC6/ODE/block ==
  Action Port : ActionPort  InitializeStates=reset
  Constant : Constant  Value=-67.39
  v : Outport
  wires:
  Constant/1 -> v/1

== system icc_lib_avg_path1_n1/ICC6/ODE/q0 ==
  reset : Inport
  vreset : Inport  Port=2
  d : Inport  Port=3
  Action Port : ActionPort  InitializeStates=reset
  Integrator1 : Integrator  ExternalReset=either  InitialConditionSource=external  InitialCondition=20
  pulse : Outport
  wires:
  Integrator1/1 -> pulse/1
  d/1 -> Integrator1/1
  reset/1 -> Integrator1/2
  vreset/1 -> Integrator1/3

== system icc_lib_avg_path1_n1/ICC6/ODE/q1 ==
  reset : Inport
  vreset : Inport  Port=2
  d : Inport  Port=3
  Action Port : ActionPort  InitializeStates=reset
  Display : Display
  Display1 : Display
  Integrator1 : Integrator  ExternalReset=either  InitialConditionSource=external  InitialCondition=20  LimitOutput=on  UpperSaturationLimit=-24.105
  Scope : Scope
  v : Outport
  wires:
  d/1 -> Integrator1/1
  Integrator1/1 -> Display/1, Scope/1, v/1
  reset/1 -> Integrator1/2
  vreset/1 -> Display1/1, Integrator1/3

== system icc_lib_avg_path1_n1/ICC6/ODE/q2 ==
  reset : Inport
  vreset : Inport  Port=2
  d : Inport  Port=3
  Action Port : ActionPort  InitializeStates=reset
  Integrator1 : Integrator  ExternalReset=either  InitialConditionSource=external  InitialCondition=20
  v : Outport
  wires:
  d/1 -> Integrator1/1
  vreset/1 -> Integrator1/3
  reset/1 -> Integrator1/2
  Integrator1/1 -> v/1

== system icc_lib_avg_path1_n1/ICC6/ODE/q3 ==
  reset : Inport
  vreset : Inport  Port=2
  d : Inport  Port=3
  theta : Inport  Port=4
  Action Port : ActionPort  InitializeStates=reset
  C : Constant  Value=-1
  Integrator1 : Integrator  ExternalReset=either  InitialConditionSource=external  InitialCondition=20  LimitOutput=on  LowerSaturationLimit=-67
  Math Function : Math  SaturateOnIntegerOverflow=on
  Product1 : Product
  Product2 : Product
  v : Outport
  wires:
  d/1 -> Integrator1/1
  Product2/1 -> Math Function/1
  C/1 -> Product2/2
  Product1/1 -> ?
  theta/1 -> Product2/1
  Math Function/1 -> Product1/2
  Integrator1/1 -> v/1
  reset/1 -> Integrator1/2
  vreset/1 -> Integrator1/3

== system icc_lib_avg_path1_n1/ICC6_egm/ODE/block ==
  Action Port : ActionPort  InitializeStates=reset
  Constant : Constant  Value=-67.39
  v : Outport
  wires:
  Constant/1 -> v/1

== system icc_lib_avg_path1_n1/ICC6_egm/ODE/q0 ==
  reset : Inport
  vreset : Inport  Port=2
  d : Inport  Port=3
  Action Port : ActionPort  InitializeStates=reset
  Integrator1 : Integrator  ExternalReset=either  InitialConditionSource=external  InitialCondition=20
  pulse : Outport
  wires:
  vreset/1 -> Integrator1/3
  reset/1 -> Integrator1/2
  d/1 -> Integrator1/1
  Integrator1/1 -> pulse/1

== system icc_lib_avg_path1_n1/ICC6_egm/ODE/q1 ==
  reset : Inport
  vreset : Inport  Port=2
  d : Inport  Port=3
  Action Port : ActionPort  InitializeStates=reset
  Display : Display
  Display1 : Display
  Integrator1 : Integrator  ExternalReset=either  InitialConditionSource=external  InitialCondition=20  LimitOutput=on  UpperSaturationLimit=-24.105
  Scope : Scope
  v : Outport
  wires:
  vreset/1 -> Integrator1/3, Display1/1
  reset/1 -> Integrator1/2
  Integrator1/1 -> v/1, Scope/1, Display/1
  d/1 -> Integrator1/1

== system icc_lib_avg_path1_n1/ICC6_egm/ODE/q2 ==
  reset : Inport
  vreset : Inport  Port=2
  d : Inport  Port=3
  Action Port : ActionPort  InitializeStates=reset
  Integrator1 : Integrator  ExternalReset=either  InitialConditionSource=external  InitialCondition=20
  v : Outport
  wires:
  Integrator1/1 -> v/1
  reset/1 -> Integrator1/2
  vreset/1 -> Integrator1/3
  d/1 -> Integrator1/1

== system icc_lib_avg_path1_n1/ICC6_egm/ODE/q3 ==
  reset : Inport
  vreset : Inport  Port=2
  d : Inport  Port=3
  theta : Inport  Port=4
  Action Port : ActionPort  InitializeStates=reset
  C : Constant  Value=-1
  Integrator1 : Integrator  ExternalReset=either  InitialConditionSource=external  InitialCondition=20  LimitOutput=on  LowerSaturationLimit=-67
  Math Function : Math  SaturateOnIntegerOverflow=on
  Product1 : Product
  Product2 : Product
  v : Outport
  wires:
  vreset/1 -> Integrator1/3
  reset/1 -> Integrator1/2
  Integrator1/1 -> v/1
  Math Function/1 -> Product1/2
  theta/1 -> Product2/1
  Product1/1 -> ?
  C/1 -> Product2/2
  Product2/1 -> Math Function/1
  d/1 -> Integrator1/1

== stateflow chart icc_lib_avg_path1_n1/ICC /Chart1 ==
  state q01
    du:
    t1=temporalCount (sec);
    pulse=-69;
  state q002
    en:m=0;
    du:
    t=temporalCount (sec);
    pulse=-67.6;
  state q001
    en:m=m+1;
    du:
    t=temporalCount (sec);
    pulse=-67.6;
  state state
    en: pulse = -67.6;
  state end
  (default) -> q002 : {m=0; t=0;}
  q001 -> q01 [order 1] : [ t >=5]{ t1=0;}
  q002 -> q001 : [t>=10]{t=0;}
  q01 -> q001 : [t1>=(0.8)]{t=0;}
  q001 -> state [order 2] : [m>6]
  state -> end
  data: m local; t local; t1 local; pulse output

== matlab function icc_lib_avg_path1_n1/ICC /MATLAB Function ==
  data: cfg output
function cfg = fcn()

%d0-o= -0.039651515;
d0= -0.042051515;
d1= 216.5795;
d2= -0.7491129;
d3= -8.890176;
%d3-1= -8.960176;

VT= -67.6;
Vm= -24.3058;
VR= -28.9622;
VF= -66.9799;

cfg=[d0,d1,d2,d3,VT,Vm,VR,VF];

end

== stateflow chart icc_lib_avg_path1_n1/ICC /Chart ==
  state wait
    entry:
    du:
    t2=temporalCount (sec);
  state q0
    en:
    q=0
  state q1
    en:
    q=1
  state q3
    en:
    q=3
  state q2
    en:
    q=2
  (default) -> wait : {t2=0;}
  wait -> q0 : [t2>=19.6]{q=0;th=0;vreset=-67.6;reset}
  q0 -> q1 [order 1] : [v<VT]/{vreset=v; th=0; Vmax=Vm;d2=d2i; reset}
  q0 -> q1 [order 2] : [gv<VT&&v>VT]{ vreset=v; th=v-VT/VF-VT; Vmax=func1(th,Vm);d2=func2(th,d2i);reset}
  q3 -> q0 : [v<VF]{vreset=v; reset}
  q1 -> q2 : [ v >Vmax ]{vreset=v; reset}
  q2 -> q3 : [v<VR]{vreset=v; reset}
  data: vmax function_output double; theta function_input; vm function_input; d2out function_output double; theta function_input; d2in function_input; v input double; q output; vreset output; gv input double; Vmm input; VT input; Vm input; VR input; VF input; th local; Vmax local; t2 local; d2i input; d2 output
  events: reset output EITHER_EDGE_EVENT
  function vmax = func1(theta,vm):
    | function vmax = func1(theta,vm)
    | 
    | m=1;
    | 
    | 
    | vmax1=Vm*exp(-m*th);
    | vmax=-25
  function d2out = func2(theta,d2in):
    | function d2out = func2(theta,d2in)
    | 
    | m=1;
    | 
    | 
    | vmax1=Vm*exp(-m*th);
    | %d2out=-0.5
    | d2out=d2in;

== matlab function icc_lib_avg_path1_n1/ICC /MATLAB Function1-freq=20  ==
  data: cfg2 output
function cfg2 = fcn()

%d0-o= -0.039651515;

%d0= -0.042051515;
%d1= 216.5795;
%d2= -0.7491129;
%d3= -8.890176;

%d3-1= -8.960176;


d0=-0.075;
d1=43.625;
d2=-0.88;
d3=-8.65;


VT= -67.6336;
Vm= -24.1075;
VR= -28.8921;
VF= -66.9586;



cfg2=[d0,d1,d2,d3,VT,Vm,VR,VF];

end

== matlab function icc_lib_avg_path1_n1/ICC /MATLAB Function-freq=24 ==
  data: cfg2 output
function cfg2 = fcn()

%d0-o= -0.039651515;

%d0= -0.042051515;
%d1= 216.5795;
%d2= -0.7491129;
%d3= -8.890176;

%d3-1= -8.960176;

%freq24
d0=-0.0381;
d1=43.568;
d2=-0.82;
d3=-4.8;


VT= -67.6336;
Vm= -24.1075;
VR= -28.8921;
VF= -66.9586;



cfg2=[d0,d1,d2,d3,VT,Vm,VR,VF];

end

== matlab function icc_lib_avg_path1_n1/ICC /MATLAB Function-freq=26-o  ==
  data: cfg2 output
function cfg2 = fcn()

%d0-o= -0.039651515;

%d0= -0.042051515;
%d1= 216.5795;
%d2= -0.7491129;
%d3= -8.890176;

%d3-1= -8.960176;

%freq26
d0=-0.053;
d1=39.5735;
d2=-0.8035;
d3=-4.69678;


VT= -67.6336;
Vm= -24.1075;
VR= -28.8921;
VF= -66.9586;



cfg2=[d0,d1,d2,d3,VT,Vm,VR,VF];

end

== matlab function icc_lib_avg_path1_n1/ICC /MATLAB Function-freq=22  ==
  data: cfg2 output
function cfg2 = fcn()

%d0-o= -0.039651515;

%d0= -0.042051515;
%d1= 216.5795;
%d2= -0.7491129;
%d3= -8.890176;

%d3-1= -8.960176;

%freq=22
d0=-0.045;
d1=43.5373;
d2=-0.835;
d3=-6.96;


VT= -67.6336;
Vm= -24.1075;
VR= -28.8921;
VF= -66.9586;



cfg2=[d0,d1,d2,d3,VT,Vm,VR,VF];

end
